simulink model "din_eml"  (R2014a)
settings: Solver=FixedStepDiscrete  SolverMode=SingleTasking  StartTime=0.0  StopTime=10.0  RelTol=1e-3
settings Model: ExtModeTrigDuration=2  Creator=gcampa  LastModifiedBy=gcampa
settings OptimizationCC: OptimizeModelRefInitCode=on  LifeSpan=1
settings DebuggingCC: UnderspecifiedInitializationDetection=Classic  SolverPrmCheckMsg=none  FrameProcessingCompatibilityMsg=error  StateNameClashWarn=warning
settings HardwareCC: ProdBitPerInt=16  ProdBitPerPointer=8  ProdIntDivRoundTo=Zero  ProdEndianess=LittleEndian  ProdWordSize=8  ProdHWDeviceType=Atmel->AVR
settings RTWCC: SystemTargetFile=realtime.tlc  GenerateMakefile=off  TemplateMakefile=realtime.tmf  Description=Run on Target Hardware  RTWVerbose=off  ProcessScript=realtime_make_rtw_hook  CustomSource=..\src\digitalio_arduino.cpp
settings STFCustomTargetCC: TargetLibSuffix=.a  GenerateSampleERTMain=on  ConcurrentExecutionCompliant=off  GeneratePreprocessorConditionals=Use local settings  ERTCustomFileBanners=on  SupportNonInlinedSFcns=off  SupportVariableSizeSignals=on  MATLABClassNameForMDSCustomization=Simulink.SoftwareTarget.ERTCustomization  GRTInterface=off  SystemTargetFile=realtime.tlc
settings ERTTargetCC: CombineOutputUpdateFcns=off  SupportContinuousTime=on  SupportVariableSizeSignals=on  ExtModeTransport=3  ExtModeMexFile=ext_serial_win32_comm  ExtModeMexArgs=0 1 9600  ERTSrcFileBannerTemplate=realtime_code_template.cgt  ERTHdrFileBannerTemplate=realtime_code_template.cgt  ERTDataSrcFileTemplate=realtime_code_template.cgt  ERTDataHdrFileTemplate=realtime_code_template.cgt  ERTCustomFileTemplate=realtime_file_process.tlc

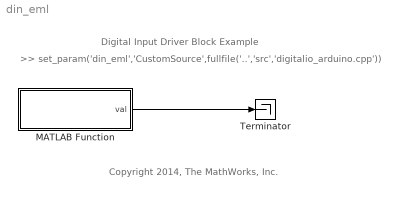
== system din_eml ==
  note: Digital Input Driver Block Example
  note: Copyright 2014, The MathWorks, Inc.
  note: >> set_param('din_eml','CustomSource',fullfile('..','src','digitalio_arduino.cpp'))
  MATLAB Function : MATLAB Function  TreatAsAtomicUnit=on  mask(Digital Read){pin=2, T=0.05}
      mask prompts: T "Sample Time"
      mask help:
      | Every time this block is executed it reads the digital value (0 or 1) of a given pin and sets it as the output of the block.
      |
      | The first parameter is the number of the pin where the digital input needs to be performed. The second parameter is the sample time.
      |
      | Note that if this block gets copied to a new model, then the file "digitalio_arduino.cpp" must be added to the CustomSource field of the new model using the "set_param" instruction. See the guide for more info.
  Terminator : Terminator
  wires:
  MATLAB Function/1(val) -> Terminator/1

== matlab function din_eml/MATLAB Function ==
  settings: updateMethod=DISCRETE  sampleTime=T
  data: pin parameter; val output
function val=digitalRead(pin)
%#codegen

persistent initflag;
val=0;

if strcmp(coder.target, 'rtw'),
    
    if isempty(initflag),
        % Initialize step
        coder.ceval('digitalIOSetup',uint8(pin),false);
        initflag = 1;
    else
        % output Step
        val=coder.ceval('readDigitalPin',uint8(pin));
    end
    
end
